simulink model "btp_rl_reward2"  (R2022a)
settings: Solver=VariableStepAuto  StartTime=0.0  StopTime=10.0  RelTol=1e-3
undefined symbols (not defined in the file or in its folder): DiscIntNeverNeededParam
libraries: simulink x3, rllib x1
settings Model: Creator=vicky  LastModifiedBy=archi

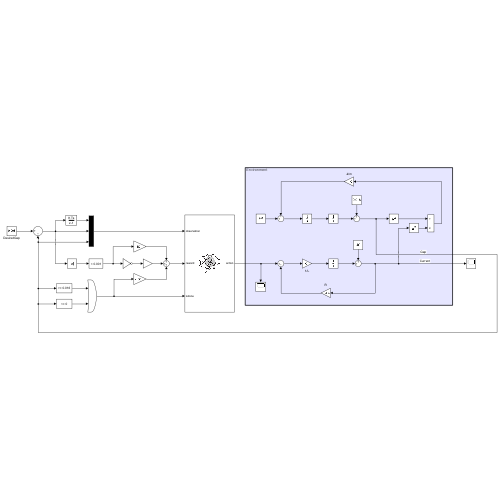
[thumbnail: Simulink's stored preview of the top-level diagram]
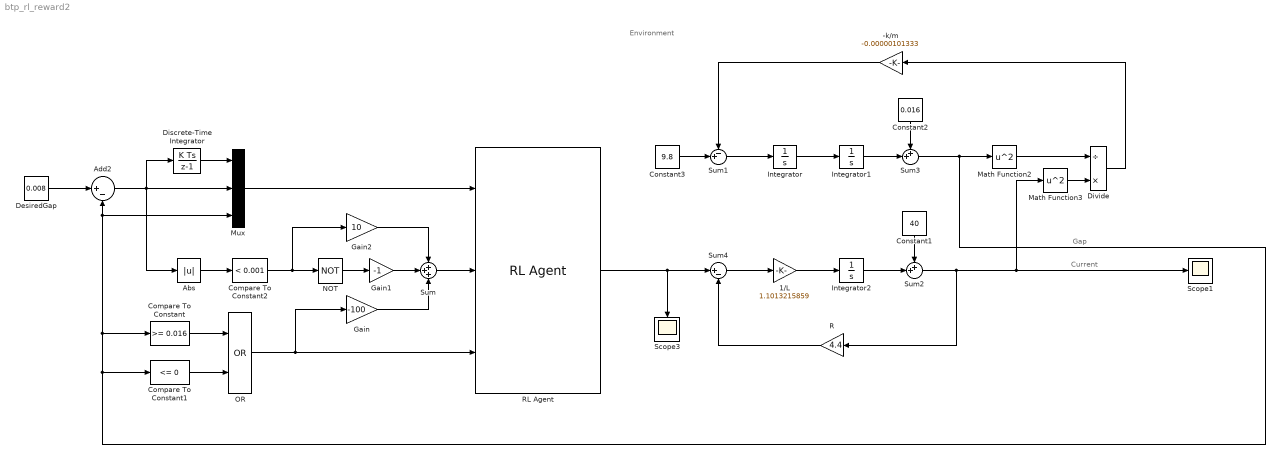
== system btp_rl_reward2 ==
  note: Gap
  note: Environment
  note: Current
  -k/m : Gain  Gain=-0.00000101333
  1/L : Gain  Gain=1.1013215859
  Abs : Abs  SaturateOnIntegerOverflow=off
  Add2 : Sum  Inputs=|+-
  Compare To Constant : simulink/Logic and Bit Operations/Compare To Constant  relop=>=  const=0.016  OutDataTypeStr=boolean
  Compare To Constant1 : simulink/Logic and Bit Operations/Compare To Constant  relop=<=  const=0  OutDataTypeStr=boolean
  Compare To Constant2 : simulink/Logic and Bit Operations/Compare To Constant  relop=<  const=0.001  OutDataTypeStr=boolean
  Constant1 : Constant  Value=40
  Constant2 : Constant  Value=0.016
  Constant3 : Constant  Value=9.8
  DesiredGap : Constant  Value=0.008
  Discrete-Time Integrator : DiscreteIntegrator  SampleTime=-1  ICPrevOutput=DiscIntNeverNeededParam  ICPrevScaledInput=DiscIntNeverNeededParam
  Divide : Product  Inputs=/*
  Gain : Gain  Gain=-100
  Gain1 : Gain  Gain=-1
  Gain2 : Gain  Gain=10
  Integrator : Integrator
  Integrator1 : Integrator
  Integrator2 : Integrator
  Math Function2 : Math  Operator=square
  Math Function3 : Math  Operator=square
  Mux : Mux  Inputs=3
  NOT : Logic  Operator=NOT  IconShape=distinctive  AllPortsSameDT=off  OutDataTypeStr=boolean
  OR : Logic  Operator=OR  IconShape=distinctive  AllPortsSameDT=off  OutDataTypeStr=boolean
  R : Gain  Gain=4.4
  RL Agent : rllib/RL Agent  Agent=rlDDPGAgent  ExternalActionAsInput=off  ProvideLastAction=off  ProvideCumRwd=off  TreatAsDirectFeedthrough=on  UseStrictObservationDataTypes=off
  Scope1 : Scope
  Scope3 : Scope
  Sum : Sum  Inputs=+++
  Sum1 : Sum  Inputs=-+|
  Sum2 : Sum  Inputs=++|
  Sum3 : Sum  Inputs=++|
  Sum4 : Sum  Inputs=|+-
  wires:
  Add2/1 -> Mux/2, Abs/1, Discrete-Time Integrator/1
  Discrete-Time Integrator/1 -> Mux/1
  Mux/1 -> RL Agent/1
  DesiredGap/1 -> Add2/1
  Compare To Constant/1 -> OR/1
  Compare To Constant1/1 -> OR/2
  OR/1 -> RL Agent/3, Gain/1
  Compare To Constant2/1 -> Gain2/1, NOT/1
  Abs/1 -> Compare To Constant2/1
  NOT/1 -> Gain1/1
  Gain/1 -> Sum/3
  Gain1/1 -> Sum/2
  Gain2/1 -> Sum/1
  Sum/1 -> RL Agent/2
  Math Function3/1 -> Divide/2
  Math Function2/1 -> Divide/1
  R/1 -> Sum4/2
  Sum1/1 -> Integrator/1
  Constant3/1 -> Sum1/2
  Integrator1/1 -> Sum3/2
  Integrator2/1 -> Sum2/2
  Integrator/1 -> Integrator1/1
  Constant1/1 -> Sum2/1
  RL Agent/1 -> Scope3/1, Sum4/1
  Sum3/1 -> Math Function2/1, Compare To Constant/1, Mux/3, Add2/2, Compare To Constant1/1
  Constant2/1 -> Sum3/1
  Sum2/1 -> R/1, Scope1/1, Math Function3/1
  1/L/1 -> Integrator2/1
  Sum4/1 -> 1/L/1
  -k/m/1 -> Sum1/1
  Divide/1 -> -k/m/1
